simulink model "step3b"  (Simulink 7.9)
settings: Solver=ode45  StartTime=0.0  StopTime=10.0  RelTol=1e-3
values from neighbouring files (symbols this model uses):
  A = [0.8 0.3; 0 -0.6]    [setup.m]
  P = dlyap(A',Q)    [setup.m]
  x0 = [1;-0.5]    [setup.m]
settings Model: Creator=aeagr  LastModifiedBy=aeagr

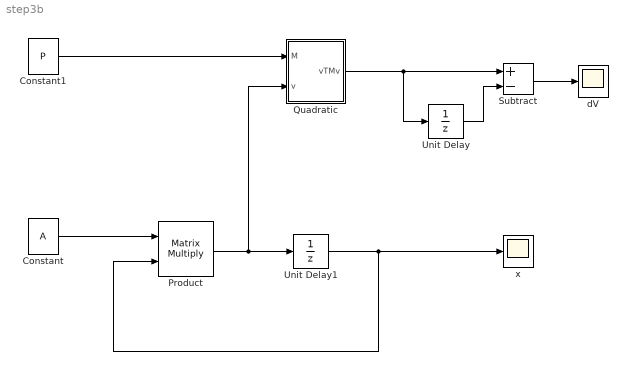
== system step3b ==
  Constant : Constant  Value=A
  Constant1 : Constant  Value=P
  Product : Product  Multiplication=Matrix(*)  RndMeth=Zero
  Quadratic : Subsystem
  Subtract : Sum  Inputs=+-
  Unit Delay : UnitDelay  X0=5
  Unit Delay1 : UnitDelay  X0=x0
  dV : Scope
  x : Scope
  wires:
  Constant/1 -> Product/1
  Product/1 -> Quadratic/2(v), Unit Delay1/1
  Unit Delay1/1 -> Product/2, x/1
  Constant1/1 -> Quadratic/1(M)
  Quadratic/1(vTMv) -> Unit Delay/1, Subtract/1
  Unit Delay/1 -> Subtract/2
  Subtract/1 -> dV/1

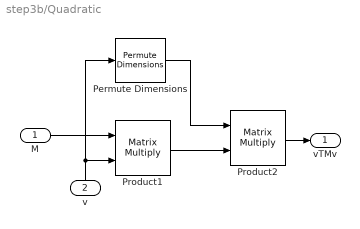
== system step3b/Quadratic ==
  M : Inport
  v : Inport  Port=2
  Permute Dimensions : PermuteDimensions
  Product1 : Product  Multiplication=Matrix(*)  RndMeth=Zero
  Product2 : Product  Multiplication=Matrix(*)  RndMeth=Zero
  vTMv : Outport
  wires:
  Product1/1 -> Product2/2
  Permute Dimensions/1 -> Product2/1
  v/1 -> Product1/2, Permute Dimensions/1
  M/1 -> Product1/1
  Product2/1 -> vTMv/1
